simulink model "sampleModel1741"  (R2023a)
settings: Solver=VariableStepAuto  StartTime=0.0  StopTime=10.0  RelTol=1e-3
libraries: hdlsllib x11, simulink x3
settings Model: Creator=user1  LastModifiedBy=user1

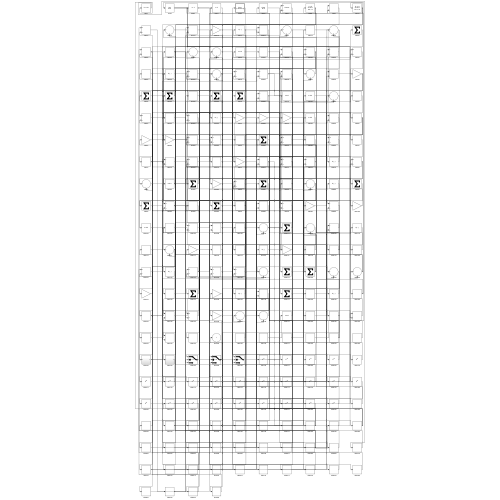
[thumbnail: Simulink's stored preview of the top-level diagram]
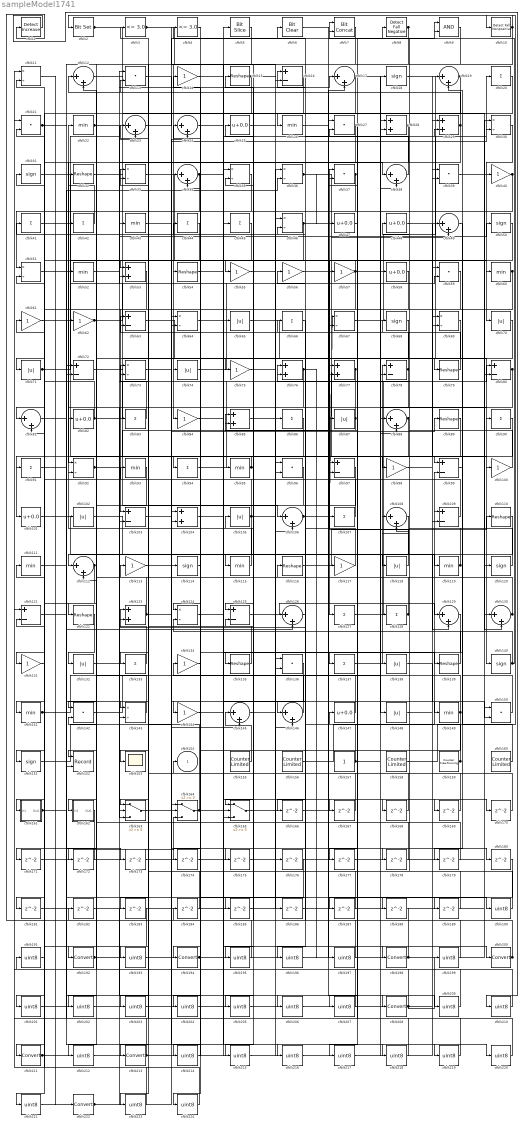
== system sampleModel1741 ==
  cfblk1 : simulink/Logic and Bit Operations/Detect Increase  vinit=0.0  OutDataTypeStr=boolean
      settings: LibrarySourceBlock=|
      | hdlsllib/Logic and Bit
      | Operations/Detect
      | Increase
  cfblk10 : hdlsllib/Logic and Bit Operations/Detect Fall Nonpositive  vinit=0  OutDataTypeStr=boolean
  cfblk{14,40,55..57,61..62,75,84,98,100,113,117,131,134,144} (16 alike) : Gain
  cfblk{25,47..48,58,82,101,147} (7 alike) : Bias  Bias=0.0  SaturateOnIntegerOverflow=off
  cfblk{65,70..71,74,87,102,105,118,132,138,148} (11 alike) : Abs  SaturateOnIntegerOverflow=off
  cfblk{16,63,72,78,80,97,99,103,109,121,125} (11 alike) : Sum  Inputs=+-
  cfblk{28..29,53,76..77,85,104,123} (8 alike) : Sum
  cfblk{12,17,19,23..24,34,38,49,81,88,106,108,112,126,129..130,145..146} (18 alike) : Sum  Inputs=|++
  cfblk{20,41..42,44..45,66,83,86,90..91,94,107,127..128,133,137} (16 alike) : Sum  Inputs=+
  cfblk{11,30,33,35..36,46,51,64,67,69,73,92,124,143} (14 alike) : Product  Inputs=*/  RndMeth=Zero  SaturateOnIntegerOverflow=on
  cfblk{15,32,54,79,89,110,116,122,135,139} (10 alike) : Reshape
  cfblk{22,26,43,52,60,93,95,111,115,119,141,149} (12 alike) : MinMax
  cfblk{18,31,50,68,114,120,140,151} (8 alike) : Signum
  cfblk{13,21,27,37,39,59,96,136,142,150} (10 alike) : DotProduct  OutDataTypeStr=Inherit: Inherit via internal rule
  cfblk152 : Record  FileSettingsInternal="{\"entries\":[{\"content\":{\"excelSettings\":{\"content\":{},\"type\":\"Streamout.ExcelSettings\"}},\"type\":\"Streamout.FileSettingStorage\",\"uuid\":\"\"}],\"packageUris\":[\"http:\\/\\/schema.mathworks.com\\/mf0\\/streamout_blocks\\/R2020a\"],\"version\":\"1.0\"}"  Layout=[1 1]  SignalsInternal="{\"entries\":[{\"content\":{\"signals\":[{\"content\":{\"blockPath\":[],\"dimensions\":[1],\"domain\":\"\",\"lineColor\":\"#a2142f\",\"plots\":[1],\"port\":1,\"signalID\":3551,\"signalName\":\"XY Graph:1\"},\"type\":\"RecordBlkView.Signal\",\"uuid\":\"\"},{\"content\":{\"blockPath\":[],\"dimensions\":[1],\"domain\":\"\",\"lineColor\":\"#139fff\",\"plots\":[1],\"port\":2,\"signalID\":3554,\"signalName\":\"XY Graph:2\"},\"type\":\"RecordBlkView.Signal\",\"uuid\":\"\"}]},\"type\":\"RecordBlkView.InputSignals\",\"uuid\":\"\"}],\"packageUris\":[\"http:\\/\\/schema.mathworks.com\\/mf0\\/streamout_blocks\\/R2020a\"],\"version\":\"1.0\"}"  VisualizationBindings="{\"xyplotplugin\":{\"info\":[{\"series\":[{\"bindingParametersList\":[{\"parameter\":\"X-Axis\",\"signalID\":3551,\"signalName\":\"XY Graph:1\"},{\"parameter\":\"Y-Axis\",\"signalID\":3554,\"signalName\":\"XY Graph:2\"}],\"seriesID\":5096}],\"subplotID\":1}]}}"  CompatibilityTag=XY  st=-1
  cfblk153 : Scope
  cfblk{155..156,158,160} (4 alike) : hdlsllib/Sources/Counter Limited  uplimit=7  tsamp=-1
  cfblk157 : Constant  SampleTime=-1
  cfblk159 : hdlsllib/Sources/Counter Free-Running  NumBits=16  tsamp=-1
  cfblk161 : Subsystem
      settings: LibrarySourceBlock=|
      | hdlsllib/Ports &
      | Subsystems/Subsystem
  cfblk162 : Subsystem
      settings: LibrarySourceBlock=|
      | hdlsllib/Ports &
      | Subsystems/Subsystem
  cfblk163 : Switch  SaturateOnIntegerOverflow=off  InputSameDT=off
  cfblk164 : Switch  SaturateOnIntegerOverflow=off  InputSameDT=off
  cfblk165 : Switch  SaturateOnIntegerOverflow=off  InputSameDT=off
  cfblk{166..189} (24 alike) : Delay  SampleTime=1
  cfblk{190..191,193,195..197,199,201..207,209..210,212,214..221,223..224} (27 alike) : DataTypeConversion  OutDataTypeStr=uint8  SaturateOnIntegerOverflow=off  RndMeth=Floor
  cfblk{192,194,198,200,208,211,213,222} (8 alike) : DataTypeConversion  SaturateOnIntegerOverflow=off  RndMeth=Floor
  cfblk2 : simulink/Logic and Bit Operations/Bit Set  iBit=0
      settings: LibrarySourceBlock=|
      | hdlsllib/Logic and Bit
      | Operations/Bit Set
  cfblk3 : hdlsllib/Logic and Bit Operations/Compare To Constant  relop=<=  const=3.0  OutDataTypeStr=boolean
  cfblk4 : hdlsllib/Logic and Bit Operations/Compare To Constant  relop=<=  const=3.0  OutDataTypeStr=boolean
  cfblk5 : hdlsllib/Logic and Bit Operations/Bit Slice  lidx=7  ridx=0
  cfblk6 : simulink/Logic and Bit Operations/Bit Clear  iBit=0
      settings: LibrarySourceBlock=|
      | hdlsllib/Logic and Bit
      | Operations/Bit Clear
  cfblk7 : hdlsllib/Logic and Bit Operations/Bit Concat  numInputs=2
  cfblk8 : hdlsllib/Logic and Bit Operations/Detect Fall Negative  vinit=0  OutDataTypeStr=boolean
  cfblk9 : Logic  AllPortsSameDT=off  OutDataTypeStr=boolean
  cfblk154 : Outport  VectorParamsAs1DForOutWhenUnconnected=off
  wires:
  cfblk72/1 -> cfblk99/1
  cfblk65/1 -> cfblk79/1
  cfblk104/1 -> cfblk200/1
  cfblk49/1 -> cfblk137/1
  cfblk11/1 -> cfblk222/1
  cfblk56/1 -> cfblk198/1
  cfblk12/1 -> cfblk55/1
  cfblk86/1 -> cfblk101/1
  cfblk110/1 -> cfblk115/1
  cfblk5/1 -> cfblk84/1
  cfblk156/1 -> cfblk99/2
  cfblk18/1 -> cfblk140/1
  cfblk98/1 -> cfblk29/1
  cfblk74/1 -> cfblk18/1
  cfblk118/1 -> cfblk37/1
  cfblk53/1 -> cfblk103/1
  cfblk137/1 -> cfblk78/1
  cfblk135/1 -> cfblk23/1
  cfblk21/1 -> cfblk151/1, cfblk143/2
  cfblk161/1(Out1) -> cfblk36/2, cfblk173/1
  cfblk34/1 -> cfblk51/1, cfblk178/1
  cfblk116/1 -> cfblk110/1
  cfblk20/1 -> cfblk26/1
  cfblk92/1 -> cfblk106/1, cfblk17/2
  cfblk122/1 -> cfblk132/1
  cfblk115/1 -> cfblk22/1
  cfblk148/1 -> cfblk19/1
  cfblk127/1 -> cfblk80/1
  cfblk15/1 -> cfblk161/1(In1), cfblk60/1
  cfblk45/1 -> cfblk211/1
  cfblk89/1 -> cfblk146/1
  cfblk32/1 -> cfblk94/1
  cfblk36/1 -> cfblk98/1, cfblk47/1
  cfblk67/1 -> cfblk20/1
  cfblk51/1 -> cfblk54/1
  cfblk125/1 -> cfblk129/1
  cfblk146/1 -> cfblk24/1
  cfblk149/1 -> cfblk25/1, cfblk224/1
  cfblk50/1 -> cfblk53/1
  cfblk95/1 -> cfblk165/1, cfblk91/1
  cfblk62/1 -> cfblk5/1, cfblk88/2
  cfblk17/1 -> cfblk90/1, cfblk122/1
  cfblk140/1 -> cfblk9/1, cfblk116/1
  cfblk28/1 -> cfblk141/1, cfblk62/1
  cfblk97/1 -> cfblk133/1
  cfblk144/1 -> cfblk65/1
  cfblk38/1 -> cfblk16/1
  cfblk33/1 -> cfblk127/1
  cfblk82/1 -> cfblk76/1, cfblk51/2, cfblk77/2
  cfblk14/1 -> cfblk139/1
  cfblk141/1 -> cfblk35/1, cfblk126/2
  cfblk35/1 -> cfblk81/1
  cfblk39/1 -> cfblk120/1
  cfblk158/1 -> cfblk10/1
  cfblk30/1 -> cfblk70/1
  cfblk87/1 -> cfblk83/1, cfblk85/2
  cfblk9/1 -> cfblk75/1
  cfblk40/1 -> cfblk81/2, cfblk77/1
  cfblk8/1 -> cfblk144/1, cfblk72/2
  cfblk37/1 -> cfblk74/1, cfblk71/1
  cfblk7/1 -> cfblk142/1
  cfblk106/1 -> cfblk67/1, cfblk169/1
  cfblk155/1 -> cfblk145/1
  cfblk151/1 -> cfblk24/2
  cfblk107/1 -> cfblk35/2
  cfblk136/1 -> cfblk164/2
  cfblk147/1 -> cfblk105/1
  cfblk160/1 -> cfblk19/2
  cfblk10/1 -> cfblk112/1, cfblk153/1, cfblk7/2, cfblk2/1
  cfblk77/1 -> cfblk152/1, cfblk183/1
  cfblk79/1 -> cfblk37/2
  cfblk6/1 -> cfblk107/1
  cfblk134/1 -> cfblk194/1
  cfblk94/1 -> cfblk49/1
  cfblk29/1 -> cfblk92/1, cfblk12/1
  cfblk108/1 -> cfblk118/1
  cfblk44/1 -> cfblk213/1
  cfblk13/1 -> cfblk145/2
  cfblk93/1 -> cfblk192/1
  cfblk157/1 -> cfblk88/1, cfblk124/2
  cfblk22/1 -> cfblk53/2, cfblk162/1(In1), cfblk38/1, cfblk202/1
  cfblk68/1 -> cfblk163/1
  cfblk150/1 -> cfblk109/1
  cfblk3/1 -> cfblk95/1, cfblk16/2
  cfblk19/1 -> cfblk152/2, cfblk185/1
  cfblk145/1 -> cfblk149/1
  cfblk112/1 -> cfblk131/1, cfblk181/1
  cfblk100/1 -> cfblk68/1
  cfblk31/1 -> cfblk126/1
  cfblk103/1 -> cfblk89/1
  cfblk101/1 -> cfblk117/1
  cfblk80/1 -> cfblk166/1, cfblk205/1
  cfblk61/1 -> cfblk17/1
  cfblk102/1 -> cfblk129/2
  cfblk52/1 -> cfblk59/2
  cfblk117/1 -> cfblk4/1
  cfblk23/1 -> cfblk9/2
  cfblk60/1 -> cfblk125/1, cfblk82/1, cfblk221/1
  cfblk54/1 -> cfblk146/2
  cfblk2/1 -> cfblk40/1, cfblk130/2, cfblk64/2
  cfblk132/1 -> cfblk50/1
  cfblk57/1 -> cfblk52/1, cfblk119/1, cfblk193/1
  cfblk121/1 -> cfblk208/1
  cfblk85/1 -> cfblk97/1
  cfblk119/1 -> cfblk76/2, cfblk13/2
  cfblk41/1 -> cfblk97/2
  cfblk48/1 -> cfblk100/1
  cfblk71/1 -> cfblk34/1, cfblk148/1
  cfblk109/1 -> cfblk31/1
  cfblk64/1 -> cfblk29/2
  cfblk120/1 -> cfblk63/1
  cfblk138/1 -> cfblk150/2
  cfblk88/1 -> cfblk135/1, cfblk163/3
  cfblk142/1 -> cfblk28/1
  cfblk126/1 -> cfblk46/2
  cfblk165/1 -> cfblk57/1
  cfblk27/1 -> cfblk143/1, cfblk207/1
  cfblk73/1 -> cfblk30/2
  cfblk75/1 -> cfblk106/2
  cfblk133/1 -> cfblk123/1
  cfblk131/1 -> cfblk61/1
  cfblk123/1 -> cfblk64/1, cfblk92/2
  cfblk130/1 -> cfblk8/1, cfblk85/1
  cfblk76/1 -> cfblk103/2, cfblk197/1
  cfblk164/1 -> cfblk33/1, cfblk189/1
  cfblk159/1 -> cfblk123/2, cfblk42/1, cfblk6/1
  cfblk105/1 -> cfblk21/2, cfblk112/2, cfblk180/1
  cfblk4/1 -> cfblk34/2
  cfblk83/1 -> cfblk73/1
  cfblk78/1 -> cfblk165/3, cfblk3/1
  cfblk139/1 -> cfblk108/2
  cfblk128/1 -> cfblk7/1, cfblk41/1
  cfblk143/1 -> cfblk102/1
  cfblk46/1 -> cfblk124/1, cfblk49/2
  cfblk63/1 -> cfblk128/1
  cfblk42/1 -> cfblk32/1
  cfblk124/1 -> cfblk167/1
  cfblk167/1 -> cfblk46/1
  cfblk26/1 -> cfblk168/1
  cfblk168/1 -> cfblk67/2
  cfblk169/1 -> cfblk63/2
  cfblk24/1 -> cfblk170/1
  cfblk170/1 -> cfblk108/1
  cfblk162/1(Out1) -> cfblk171/1
  cfblk171/1 -> cfblk80/2
  cfblk16/1 -> cfblk172/1
  cfblk172/1 -> cfblk164/3
  cfblk173/1 -> cfblk59/1
  cfblk114/1 -> cfblk174/1
  cfblk174/1 -> cfblk150/1
  cfblk163/1 -> cfblk175/1
  cfblk175/1 -> cfblk109/2
  cfblk55/1 -> cfblk176/1
  cfblk47/1 -> cfblk177/1
  cfblk177/1 -> cfblk28/2
  cfblk178/1 -> cfblk142/2
  cfblk99/1 -> cfblk179/1
  cfblk179/1 -> cfblk165/2
  cfblk181/1 -> cfblk30/1
  cfblk184/1 -> cfblk33/2
  cfblk185/1 -> cfblk136/2
  cfblk25/1 -> cfblk186/1
  cfblk186/1 -> cfblk78/2
  cfblk58/1 -> cfblk187/1
  cfblk187/1 -> cfblk164/1
  cfblk91/1 -> cfblk188/1
  cfblk188/1 -> cfblk1/1
  cfblk189/1 -> cfblk73/2
  cfblk111/1 -> cfblk190/1
  cfblk190/1 -> cfblk48/1
  cfblk191/1 -> cfblk111/1
  cfblk192/1 -> cfblk130/1, cfblk58/1
  cfblk193/1 -> cfblk93/1
  cfblk194/1 -> cfblk38/2, cfblk14/1
  cfblk59/1 -> cfblk195/1
  cfblk195/1 -> cfblk134/1
  cfblk66/1 -> cfblk196/1
  cfblk196/1 -> cfblk27/1
  cfblk197/1 -> cfblk66/1
  cfblk198/1 -> cfblk27/2, cfblk125/2, cfblk154/1
  cfblk199/1 -> cfblk56/1
  cfblk200/1 -> cfblk184/1, cfblk36/1, cfblk15/1
  cfblk183/1 -> cfblk201/1
  cfblk201/1 -> cfblk104/1
  cfblk202/1 -> cfblk104/2
  cfblk96/1 -> cfblk203/1
  cfblk203/1 -> cfblk39/2
  cfblk176/1 -> cfblk204/1
  cfblk204/1 -> cfblk96/1
  cfblk205/1 -> cfblk96/2
  cfblk182/1 -> cfblk206/1
  cfblk206/1 -> cfblk39/1
  cfblk207/1 -> cfblk182/1
  cfblk208/1 -> cfblk199/1, cfblk12/2, cfblk13/1, cfblk87/1
  cfblk166/1 -> cfblk209/1
  cfblk209/1 -> cfblk121/1
  cfblk1/1 -> cfblk210/1
  cfblk210/1 -> cfblk121/2
  cfblk211/1 -> cfblk23/2, cfblk136/1
  cfblk70/1 -> cfblk212/1
  cfblk212/1 -> cfblk45/1
  cfblk213/1 -> cfblk191/1, cfblk72/1, cfblk86/1
  cfblk129/1 -> cfblk214/1
  cfblk214/1 -> cfblk44/1
  cfblk69/1 -> cfblk215/1
  cfblk215/1 -> cfblk138/1
  cfblk81/1 -> cfblk216/1
  cfblk216/1 -> cfblk69/1
  cfblk180/1 -> cfblk217/1
  cfblk217/1 -> cfblk69/2
  cfblk113/1 -> cfblk218/1
  cfblk218/1 -> cfblk21/1
  cfblk84/1 -> cfblk219/1
  cfblk219/1 -> cfblk113/1
  cfblk43/1 -> cfblk220/1
  cfblk220/1 -> cfblk147/1
  cfblk221/1 -> cfblk43/1
  cfblk222/1 -> cfblk163/2, cfblk114/1
  cfblk90/1 -> cfblk223/1
  cfblk223/1 -> cfblk11/1
  cfblk224/1 -> cfblk11/2

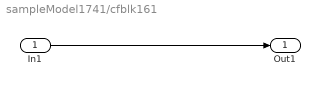
== system sampleModel1741/cfblk161 ==
  In1 : Inport
  Out1 : Outport
  wires:
  In1/1 -> Out1/1

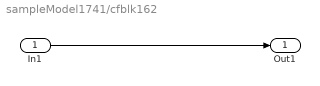
== system sampleModel1741/cfblk162 ==
  In1 : Inport
  Out1 : Outport
  wires:
  In1/1 -> Out1/1
